simulink model "CMU_BORG_AplysiaModularNeuromechanics"  (R2024a)
settings: Solver=ode23  StartTime=0.0  StopTime=tend  FixedStep=0.001  MaxStep=0.1  RelTol=0.00001  AbsTol=0.0001
values from neighbouring files (symbols this model uses):
  B20_0 = 0    [ParameterRecalculation.m]    (also in ReferenceGeometry_and_Initialization.m)
  B31B32_0 = 0    [GetSteadyState.m]    (also in ParameterRecalculation.m = 1; ReferenceGeometry_and_Initialization.m = 1; VaryingSeaweedStrength.m = 1)
  B38_0 = 0    [ParameterRecalculation.m]    (also in ReferenceGeometry_and_Initialization.m)
  B40B30_0 = 0    [ParameterRecalculation.m]    (also in ReferenceGeometry_and_Initialization.m)
  B40B30_offTime_0 = 0    [ParameterRecalculation.m]    (also in ReferenceGeometry_and_Initialization.m)
  B43B45_0 = 0    [ParameterRecalculation.m]    (also in ReferenceGeometry_and_Initialization.m)
  B4B5_0 = 0    [ParameterRecalculation.m]    (also in ReferenceGeometry_and_Initialization.m)
  B64_0 = 1    [GetSteadyState.m]    (also in ParameterRecalculation.m = 0; ReferenceGeometry_and_Initialization.m = 0; VaryingSeaweedStrength.m = 0)
  B6B9B3_0 = 1    [GetSteadyState.m]    (also in ParameterRecalculation.m = 0; ReferenceGeometry_and_Initialization.m = 0; VaryingSeaweedStrength.m = 0)
  B7_0 = 0    [ParameterRecalculation.m]    (also in ReferenceGeometry_and_Initialization.m)
  B8_0 = 0    [ParameterRecalculation.m]    (also in ReferenceGeometry_and_Initialization.m)
  C1_0 = 0    [ParameterRecalculation.m]    (also in ReferenceGeometry_and_Initialization.m)
  C2_0 = 0    [ParameterRecalculation.m]    (also in ReferenceGeometry_and_Initialization.m)
  C6_0 = 0    [ParameterRecalculation.m]    (also in ReferenceGeometry_and_Initialization.m)
  C_theta = C_xg/(2*pi)    [ParameterRecalculation.m]    (also in ReferenceGeometry_and_Initialization.m = 0.000813600069086)
  C_xd = C_xg    [ParameterRecalculation.m]    (also in ReferenceGeometry_and_Initialization.m = 0.005112)
  C_xg = (1/inv_C(kk))*time_scaler*force_scaler    [DampingParameterConvergence.m]    (also in ReferenceGeometry_and_Initialization.m = 0.005112)
  C_xv = C_xd    [ParameterRecalculation.m]    (also in ReferenceGeometry_and_Initialization.m = 0.005112)
  C_yg = C_xg    [ParameterRecalculation.m]    (also in ReferenceGeometry_and_Initialization.m = 0.005112)
  CBI2_0 = 0    [ParameterRecalculation.m]    (also in ReferenceGeometry_and_Initialization.m)
  CBI3_0 = 0    [GetSteadyState.m]    (also in ParameterRecalculation.m = 1; ReferenceGeometry_and_Initialization.m = 1; VaryingSeaweedStrength.m = 1)
  CBI3_refractory_0 = 0    [ParameterRecalculation.m]    (also in ReferenceGeometry_and_Initialization.m)
  CBI3_stimOFF_0 = 0    [ParameterRecalculation.m]    (also in ReferenceGeometry_and_Initialization.m)
  CBI3_stimON_0 = 0    [ParameterRecalculation.m]    (also in ReferenceGeometry_and_Initialization.m)
  CBI4_0 = 0    [ParameterRecalculation.m]    (also in ReferenceGeometry_and_Initialization.m)
  E1_params = [AE10,TE10,tau_E1,L0_E1,Lmax_E1]    [ParameterRecalculation.m]    (also in ReferenceGeometry_and_Initialization.m)
  E2_params = [AE20,TE20,tau_E2,L0_E2,Lmax_E2]    [ParameterRecalculation.m]    (also in ReferenceGeometry_and_Initialization.m)
  E6_params = [AE60,TE60,tau_E6,L0_E6,Lmax_E6]    [ParameterRecalculation.m]    (also in ReferenceGeometry_and_Initialization.m)
  FE1_max = force_scaler*0.2    [ParameterRecalculation.m]    (also in ReferenceGeometry_and_Initialization.m = 0.048)
  FE2_max = FE1_max    [ParameterRecalculation.m]    (also in ReferenceGeometry_and_Initialization.m = 0.048)
  FE6_max = FE1_max    [ParameterRecalculation.m]    (also in ReferenceGeometry_and_Initialization.m = 0.048)
  FHinge_max = force_scaler*0.292    [ParameterRecalculation.m]    (also in ReferenceGeometry_and_Initialization.m = 0.07008)
  FI1d_max = force_scaler*3.2    [ParameterRecalculation.m]    (also in ReferenceGeometry_and_Initialization.m = 0.768)
  FI1v_max = FI1d_max    [ParameterRecalculation.m]    (also in ReferenceGeometry_and_Initialization.m = 0.768)
  FI2_max = force_scaler*1    [ParameterRecalculation.m]    (also in ReferenceGeometry_and_Initialization.m = 0.24)
  FI3_ant_max = force_scaler*0.1    [ParameterRecalculation.m]    (also in ReferenceGeometry_and_Initialization.m = 0.024)
  FI3_max = force_scaler*3    [ParameterRecalculation.m]    (also in ReferenceGeometry_and_Initialization.m = 0.72)
  FI4_max = force_scaler*0.9    [ParameterRecalculation.m]    (also in ReferenceGeometry_and_Initialization.m = 0.216)
  fixation_type = 0    [GetSteadyState.m]    (also in ModelController.m; VaryingSeaweedStrength.m)
  grasperR = 1    [ReferenceGeometry_and_Initialization.m]
  H_lumen = mean([L_jaw,L_LG]) / R_ref    [ReferenceGeometry_and_Initialization.m]
  Hinge_params = [A_hinge0,T_hinge0,tau_hinge,L0_hinge,Lmax_hinge]    [ParameterRecalculation.m]    (also in ReferenceGeometry_and_Initialization.m)
  I1d_params = [AI1d0,TI1d0,tau_I1d,L0_I1d,Lmax_I1d]    [ParameterRecalculation.m]    (also in ReferenceGeometry_and_Initialization.m)
  I1v_params = [AI1v0,TI1v0,tau_I1v,L0_I1v,Lmax_I1v]    [ParameterRecalculation.m]    (also in ReferenceGeometry_and_Initialization.m)
  I2_params = [AI20,TI20,tau_I2_ingestive,tau_I2_egestive,L0_I2,Lmax_I2]    [ParameterRecalculation.m]    (also in ReferenceGeometry_and_Initialization.m)
  I3_params = [AI30,TI30,tau_I3]    [ParameterRecalculation.m]    (also in ReferenceGeometry_and_Initialization.m)
  I3ant_params = [AI3_ant0,TI3_ant0,tau_I3ant]    [ParameterRecalculation.m]    (also in ReferenceGeometry_and_Initialization.m)
  I4_params = [AI40,TI40,tau_I4]    [ParameterRecalculation.m]    (also in ReferenceGeometry_and_Initialization.m)
  K_const = force_scaler*0.5    [ParameterRecalculation.m]    (also in ReferenceGeometry_and_Initialization.m = 0.12)
  K_Eso = force_scaler*0.01    [ParameterRecalculation.m]    (also in ReferenceGeometry_and_Initialization.m = 0.0024)
  K_H = force_scaler*2    [ParameterRecalculation.m]    (also in ReferenceGeometry_and_Initialization.m = 0.48)
  L0_eso = abs(xd0)    [ReferenceGeometry_and_Initialization.m]
  L0_H = 0    [ReferenceGeometry_and_Initialization.m]
  L0_I1d = L1d0    [ParameterRecalculation.m]    (also in ReferenceGeometry_and_Initialization.m)
  L0_I1v = L1v0    [ParameterRecalculation.m]    (also in ReferenceGeometry_and_Initialization.m)
  L_head = 0.82*tracing_scale_factor    [ReferenceGeometry_and_Initialization.m]
  MCC_0 = 1    [DampingParameterConvergence.m]    (also in ModelController.m; ParameterRecalculation.m = 0; ReferenceGeometry_and_Initialization.m = 0)
  params = param_vec    [ParameterRecalculation.m]    (also in ReferenceGeometry_and_Initialization.m)
  seaweed_strength = 1e6    (= 1000000)    [ModelController.m]    (also in VaryingSeaweedStrength.m = seaweed_strength_vec(ind))
  sens_chemical_lips = 0    [GetSteadyState.m]    (also in ModelController.m = 1; VaryingSeaweedStrength.m = 1)
  sens_mechanical_grasper = 1    [GetSteadyState.m]    (also in ModelController.m = 0; VaryingSeaweedStrength.m)
  sens_mechanical_lips = 1    [GetSteadyState.m]    (also in ModelController.m; VaryingSeaweedStrength.m)
  t_switch_chem_lips = 1e6    (= 1000000)    [GetSteadyState.m]    (also in ModelController.m = 54; VaryingSeaweedStrength.m)
  t_switch_fixation = 1e6    (= 1000000)    [GetSteadyState.m]    (also in ModelController.m = 30; VaryingSeaweedStrength.m = 4)
  t_switch_mech_grasp = 1e6    (= 1000000)    [GetSteadyState.m]    (also in ModelController.m = 10; VaryingSeaweedStrength.m)
  t_switch_mech_lips = 1e6    (= 1000000)    [GetSteadyState.m]    (also in ModelController.m; VaryingSeaweedStrength.m)
  theta_fg = buccal_mass_data(7)    [PlotModel.m]    (also in ReferenceGeometry_and_Initialization.m = -(head_outline{4,"Angle"} - head_outline{3,"Angle"})*(pi/180)
  theta_g0 = (180-(head_outline{3,"Angle"} + rot_global +5))*(pi/180)    [ReferenceGeometry_and_Initialization.m]
  theta_H = buccal_mass_data(6)    [PlotModel.m]    (also in ReferenceGeometry_and_Initialization.m = pi + theta_H_tilde - theta_g0)
  time_scaler = 1    [DampingParameterConvergence.m]    (also in ReferenceGeometry_and_Initialization.m = 1.065)
  ukg = 0.95*usg    (= 0.95)    [ParameterRecalculation.m]    (also in ReferenceGeometry_and_Initialization.m)
  ukh = 0.75*ush    (= 0.75)    [ParameterRecalculation.m]    (also in ReferenceGeometry_and_Initialization.m)
  usg = 1    [ParameterRecalculation.m]    (also in ReferenceGeometry_and_Initialization.m)
  ush = 1    [ParameterRecalculation.m]    (also in ReferenceGeometry_and_Initialization.m)
  xd0 = L_head - L1d0    [ReferenceGeometry_and_Initialization.m]
  xg0 = L_head + L_CG * cosd(a_CG) + 0.3    [ReferenceGeometry_and_Initialization.m]
  xh0 = 0    [ReferenceGeometry_and_Initialization.m]
  xv0 = L_head - L1v0    [ReferenceGeometry_and_Initialization.m]
  yg0 = L_CG * sind(a_CG) + 0.4    [ReferenceGeometry_and_Initialization.m]
(part 3 of 4)

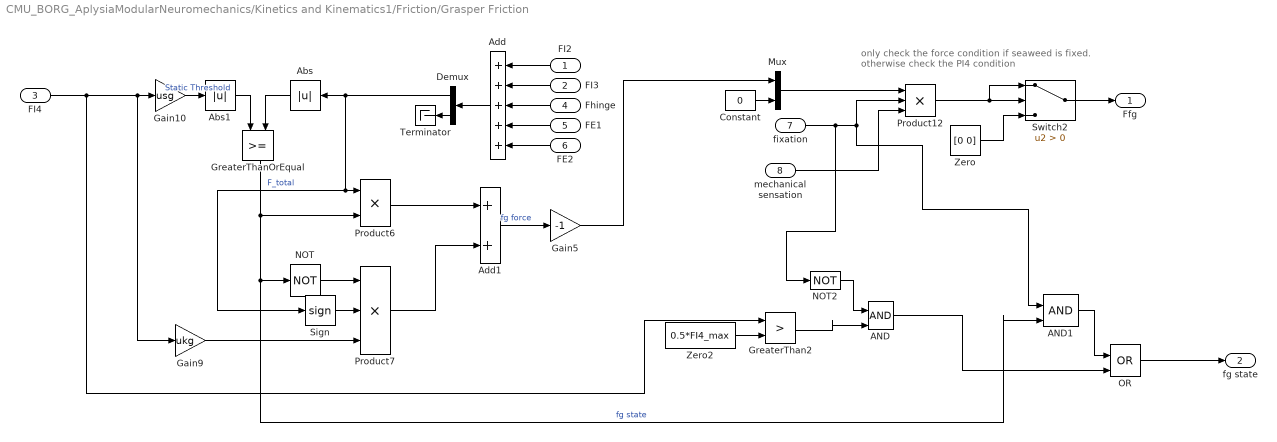
== system CMU_BORG_AplysiaModularNeuromechanics/Kinetics and Kinematics1/Friction/Grasper Friction ==
  note: only check the force condition if seaweed is fixed.
      | otherwise check the PI4 condition
  FI2 : Inport
  FI3 : Inport  Port=2
  FI4 : Inport  Port=3
  Fhinge : Inport  Port=4
  FE1 : Inport  Port=5
  FE2 : Inport  Port=6
  fixation : Inport  Port=7
  mechanical sensation : Inport  Port=8
  AND : Logic  IconShape=distinctive  AllPortsSameDT=off  OutDataTypeStr=boolean
  AND1 : Logic  IconShape=distinctive  AllPortsSameDT=off  OutDataTypeStr=boolean
  Abs : Abs  ZeroCross=off  SaturateOnIntegerOverflow=off
  Abs1 : Abs  ZeroCross=off  SaturateOnIntegerOverflow=off
  Add : Sum  Inputs=+++++
  Add1 : Sum
  Constant : Constant  Value=0
  Demux : Demux  Outputs=2
  Gain10 : Gain  Gain=usg
  Gain5 : Gain  Gain=-1
  Gain9 : Gain  Gain=ukg
  GreaterThan2 : RelationalOperator  Operator=>  OutDataTypeStr=boolean  RndMeth=Simplest  InputSameDT=off
  GreaterThanOrEqual : RelationalOperator  OutDataTypeStr=boolean  ZeroCross=off  RndMeth=Simplest  InputSameDT=off
  Mux : Mux  Inputs=2
  NOT : Logic  Operator=NOT  IconShape=distinctive  AllPortsSameDT=off  OutDataTypeStr=boolean
  NOT2 : Logic  Operator=NOT  IconShape=distinctive  AllPortsSameDT=off  OutDataTypeStr=boolean
  OR : Logic  Operator=OR  IconShape=distinctive  AllPortsSameDT=off  OutDataTypeStr=boolean
  Product12 : Product  Inputs=3
  Product6 : Product
  Product7 : Product  Inputs=3
  Sign : Signum  ZeroCross=off
  Switch2 : Switch  Criteria=u2 > Threshold  SaturateOnIntegerOverflow=off  InputSameDT=off
  Terminator : Terminator
  Zero : Constant  Value=[0 0]  OutDataTypeStr=Inherit: Inherit via back propagation
  Zero2 : Constant  Value=0.5*FI4_max  OutDataTypeStr=Inherit: Inherit via back propagation
  Ffg : Outport
  fg state : Outport  Port=2
  wires:
  Product6/1 -> Add1/1
  Abs1/1 -> GreaterThanOrEqual/1
  NOT/1 -> Product7/1
  Gain9/1 -> Product7/3
  Product7/1 -> Add1/2
  Sign/1 -> Product7/2
  Add1/1 -> Gain5/1  "fg force"
  Abs/1 -> GreaterThanOrEqual/2
  FI4/1 -> GreaterThan2/1, Gain10/1, Gain9/1
  GreaterThanOrEqual/1 -> AND1/2, NOT/1, Product6/2  "fg state"
  Gain10/1 -> Abs1/1  "Static Threshold"
  FI2/1 -> Add/1
  FE2/1 -> Add/5
  FE1/1 -> Add/4
  Fhinge/1 -> Add/3
  FI3/1 -> Add/2
  Add/1 -> Demux/1
  Demux/1 -> Sign/1, Product6/1, Abs/1  "F_total"
  Demux/2 -> Terminator/1
  Constant/1 -> Mux/2
  mechanical sensation/1 -> Product12/3
  fixation/1 -> NOT2/1, AND1/1, Product12/2
  Mux/1 -> Product12/1
  Product12/1 -> Switch2/2, Switch2/1
  Zero/1 -> Switch2/3
  Switch2/1 -> Ffg/1
  Gain5/1 -> Mux/1
  OR/1 -> fg state/1
  AND/1 -> OR/2
  Zero2/1 -> GreaterThan2/2
  AND1/1 -> OR/1
  GreaterThan2/1 -> AND/2
  NOT2/1 -> AND/1

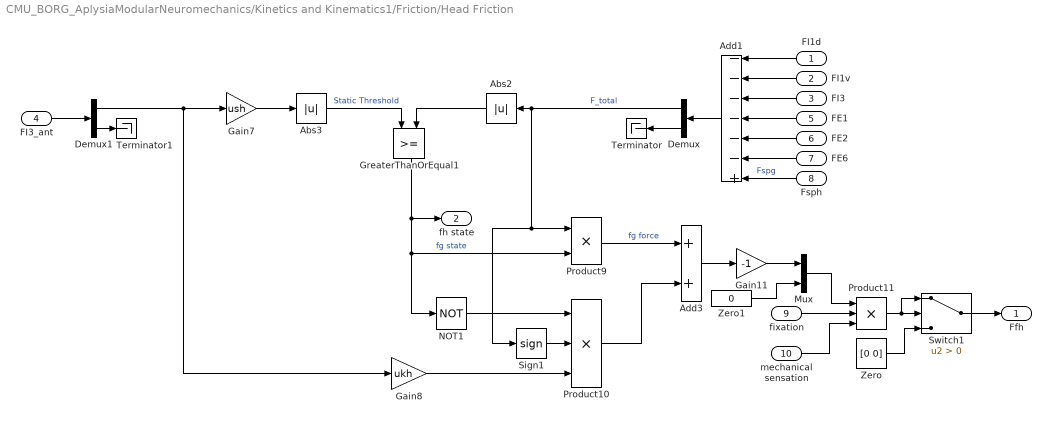
== system CMU_BORG_AplysiaModularNeuromechanics/Kinetics and Kinematics1/Friction/Head Friction ==
  FI1d : Inport
  FI1v : Inport  Port=2
  FI3 : Inport  Port=3
  FI3_ant : Inport  Port=4
  FE1 : Inport  Port=5
  FE2 : Inport  Port=6
  FE6 : Inport  Port=7
  Fsph : Inport  Port=8
  fixation : Inport  Port=9
  mechanical sensation : Inport  Port=10
  Abs2 : Abs  ZeroCross=off  SaturateOnIntegerOverflow=off
  Abs3 : Abs  ZeroCross=off  SaturateOnIntegerOverflow=off
  Add1 : Sum  Inputs=------+
  Add3 : Sum
  Demux : Demux  Outputs=2
  Demux1 : Demux  Outputs=2
  Gain11 : Gain  Gain=-1
  Gain7 : Gain  Gain=ush
  Gain8 : Gain  Gain=ukh
  GreaterThanOrEqual1 : RelationalOperator  OutDataTypeStr=boolean  ZeroCross=off  RndMeth=Simplest  InputSameDT=off
  Mux : Mux  Inputs=2
  NOT1 : Logic  Operator=NOT  IconShape=distinctive  AllPortsSameDT=off  OutDataTypeStr=boolean
  Product10 : Product  Inputs=3
  Product11 : Product  Inputs=3
  Product9 : Product
  Sign1 : Signum  ZeroCross=off
  Switch1 : Switch  Criteria=u2 > Threshold  SaturateOnIntegerOverflow=off  InputSameDT=off
  Terminator : Terminator
  Terminator1 : Terminator
  Zero : Constant  Value=[0 0]  OutDataTypeStr=Inherit: Inherit via back propagation
  Zero1 : Constant  Value=0  OutDataTypeStr=Inherit: Inherit via back propagation
  Ffh : Outport
  fh state : Outport  Port=2
  wires:
  Add3/1 -> Gain11/1
  Gain8/1 -> Product10/3
  Product10/1 -> Add3/2
  Gain7/1 -> Abs3/1
  NOT1/1 -> Product10/1
  Sign1/1 -> Product10/2
  Abs2/1 -> GreaterThanOrEqual1/2
  FI1d/1 -> Add1/1
  FI1v/1 -> Add1/2
  FI3/1 -> Add1/3
  FE1/1 -> Add1/4
  FE2/1 -> Add1/5
  FE6/1 -> Add1/6
  Fsph/1 -> Add1/7  "Fspg"
  Add1/1 -> Demux/1
  Demux/2 -> Terminator/1
  fixation/1 -> Product11/2
  mechanical sensation/1 -> Product11/3
  Product11/1 -> Switch1/2, Switch1/1
  Zero/1 -> Switch1/3
  Product9/1 -> Add3/1  "fg force"
  Abs3/1 -> GreaterThanOrEqual1/1  "Static Threshold"
  GreaterThanOrEqual1/1 -> NOT1/1, Product9/2, fh state/1  "fg state"
  Demux/1 -> Sign1/1, Product9/1, Abs2/1  "F_total"
  Demux1/1 -> Gain8/1, Gain7/1
  FI3_ant/1 -> Demux1/1
  Demux1/2 -> Terminator1/1
  Gain11/1 -> Mux/1
  Mux/1 -> Product11/1
  Zero1/1 -> Mux/2
  Switch1/1 -> Ffh/1

== system CMU_BORG_AplysiaModularNeuromechanics/Kinetics and Kinematics1/Kinematics (Circular Odontophore)/E1 Length//Angle ==
  Anchor : Inport
  Attachment : Inport  Port=2
  Add : Sum
  Atan : Trigonometry  Operator=atan
  Demux1 : Demux  Outputs=2
  Demux3 : Demux  Outputs=2
  Divide : Product  Inputs=/*
  Sqrt : Sqrt
  Square : Math  Operator=square
  Sum3 : Sum  Inputs=+-|
  L : Outport
  phi : Outport  Port=2
  wires:
  Add/1 -> Sqrt/1
  Square/1 -> Demux3/1
  Demux3/2 -> Add/2
  Demux3/1 -> Add/1
  Sum3/1 -> Demux1/1, Square/1
  Anchor/1 -> Sum3/1
  Attachment/1 -> Sum3/2
  Sqrt/1 -> L/1
  Demux1/1 -> Divide/1
  Demux1/2 -> Divide/2
  Divide/1 -> Atan/1
  Atan/1 -> phi/1

== system CMU_BORG_AplysiaModularNeuromechanics/Kinetics and Kinematics1/Kinematics (Circular Odontophore)/E2 Length//Angle ==
  Anchor : Inport
  Attachment : Inport  Port=2
  Add : Sum
  Atan : Trigonometry  Operator=atan
  Demux1 : Demux  Outputs=2
  Demux3 : Demux  Outputs=2
  Divide : Product  Inputs=/*
  Sqrt : Sqrt
  Square : Math  Operator=square
  Sum3 : Sum  Inputs=+-|
  L : Outport
  phi : Outport  Port=2
  wires:
  Atan/1 -> phi/1
  Divide/1 -> Atan/1
  Demux1/2 -> Divide/2
  Demux1/1 -> Divide/1
  Sqrt/1 -> L/1
  Attachment/1 -> Sum3/2
  Anchor/1 -> Sum3/1
  Sum3/1 -> Square/1, Demux1/1
  Demux3/1 -> Add/1
  Demux3/2 -> Add/2
  Square/1 -> Demux3/1
  Add/1 -> Sqrt/1

== system CMU_BORG_AplysiaModularNeuromechanics/Kinetics and Kinematics1/Kinematics (Circular Odontophore)/E6 Length//Angle ==
  Anchor : Inport  PortDimensions=2
  Attachment : Inport  Port=2
  Add : Sum
  Atan : Trigonometry  Operator=atan
  Demux1 : Demux  Outputs=2
  Demux3 : Demux  Outputs=2
  Divide : Product  Inputs=/*
  Sqrt : Sqrt
  Square : Math  Operator=square
  Sum3 : Sum  Inputs=+-|
  L : Outport
  phi : Outport  Port=2
  wires:
  Atan/1 -> phi/1
  Divide/1 -> Atan/1
  Demux1/2 -> Divide/2
  Demux1/1 -> Divide/1
  Sqrt/1 -> L/1
  Attachment/1 -> Sum3/2
  Anchor/1 -> Sum3/1
  Sum3/1 -> Square/1, Demux1/1
  Demux3/1 -> Add/1
  Demux3/2 -> Add/2
  Square/1 -> Demux3/1
  Add/1 -> Sqrt/1

== system CMU_BORG_AplysiaModularNeuromechanics/Kinetics and Kinematics1/Kinematics (Circular Odontophore)/Hinge Length//Angle ==
  Attachment : Inport
  Anchor : Inport  Port=2
  Add : Sum
  Atan : Trigonometry  Operator=atan
  Constant : Constant  Value=0
  Demux1 : Demux  Outputs=2
  Demux3 : Demux  Outputs=2
  Divide : Product  Inputs=/*
  Sqrt : Sqrt
  Square : Math  Operator=square
  Sum3 : Sum  Inputs=+-|
  L : Outport
  phi : Outport  Port=2
  wires:
  Divide/1 -> Atan/1
  Demux1/2 -> Divide/2
  Demux1/1 -> Divide/1
  Attachment/1 -> Sum3/2
  Anchor/1 -> Sum3/1
  Sum3/1 -> Square/1, Demux1/1
  Demux3/1 -> Add/1
  Square/1 -> Demux3/1
  Add/1 -> Sqrt/1
  Sqrt/1 -> L/1
  Atan/1 -> phi/1
  Constant/1 -> Add/2

== system CMU_BORG_AplysiaModularNeuromechanics/Kinetics and Kinematics1/Kinematics (Circular Odontophore)/I1d Length//Angle ==
  Anchor : Inport
  Attachment : Inport  Port=2
  Add : Sum
  Atan : Trigonometry  Operator=atan
  Demux1 : Demux  Outputs=2
  Demux3 : Demux  Outputs=2
  Divide : Product  Inputs=/*
  Sqrt : Sqrt
  Square : Math  Operator=square
  Sum3 : Sum  Inputs=+-|
  L : Outport
  phi : Outport  Port=2
  wires:
  Atan/1 -> phi/1
  Divide/1 -> Atan/1
  Demux1/2 -> Divide/2
  Demux1/1 -> Divide/1
  Sqrt/1 -> L/1
  Attachment/1 -> Sum3/2
  Anchor/1 -> Sum3/1
  Sum3/1 -> Square/1, Demux1/1
  Demux3/1 -> Add/1
  Demux3/2 -> Add/2
  Square/1 -> Demux3/1
  Add/1 -> Sqrt/1

== system CMU_BORG_AplysiaModularNeuromechanics/Kinetics and Kinematics1/Kinematics (Circular Odontophore)/I1v Length//Angle ==
  Anchor : Inport
  Attachment : Inport  Port=2
  Add : Sum
  Atan : Trigonometry  Operator=atan
  Demux1 : Demux  Outputs=2
  Demux3 : Demux  Outputs=2
  Divide : Product  Inputs=/*
  Sqrt : Sqrt
  Square : Math  Operator=square
  Sum3 : Sum  Inputs=+-|
  L : Outport
  phi : Outport  Port=2
  wires:
  Add/1 -> Sqrt/1
  Square/1 -> Demux3/1
  Demux3/2 -> Add/2
  Demux3/1 -> Add/1
  Sum3/1 -> Demux1/1, Square/1
  Anchor/1 -> Sum3/1
  Attachment/1 -> Sum3/2
  Sqrt/1 -> L/1
  Demux1/1 -> Divide/1
  Demux1/2 -> Divide/2
  Divide/1 -> Atan/1
  Atan/1 -> phi/1

== system CMU_BORG_AplysiaModularNeuromechanics/Kinetics and Kinematics1/Kinematics (Circular Odontophore)/I2d Length//Angle ==
  Anchor : Inport
  Attachment : Inport  Port=2
  Add : Sum
  Atan : Trigonometry  Operator=atan
  Demux1 : Demux  Outputs=2
  Demux3 : Demux  Outputs=2
  Divide : Product  Inputs=/*
  Sqrt : Sqrt
  Square : Math  Operator=square
  Sum3 : Sum  Inputs=+-|
  L : Outport
  phi : Outport  Port=2
  wires:
  Atan/1 -> phi/1
  Divide/1 -> Atan/1
  Demux1/2 -> Divide/2
  Demux1/1 -> Divide/1
  Sqrt/1 -> L/1
  Attachment/1 -> Sum3/2
  Anchor/1 -> Sum3/1
  Sum3/1 -> Square/1, Demux1/1
  Demux3/1 -> Add/1
  Demux3/2 -> Add/2
  Square/1 -> Demux3/1
  Add/1 -> Sqrt/1

== system CMU_BORG_AplysiaModularNeuromechanics/Kinetics and Kinematics1/Kinematics (Circular Odontophore)/I2v Length//Angle1 ==
  note: Switch accounts for when hinge is inside odontophore. If inside,
      | state that the I2 angle is 0 relative to the horizontal.
  Attachment : Inport
  Anchor : Inport  Port=2
  Add : Sum
  Atan : Trigonometry  Operator=atan
  Constant : Constant  Value=0
  Demux1 : Demux  Outputs=2
  Demux3 : Demux  Outputs=2
  Divide : Product  Inputs=/*
  Sqrt : Sqrt
  Square : Math  Operator=square
  Sum3 : Sum  Inputs=+-|
  Switch : Switch  Criteria=u2 > Threshold  SaturateOnIntegerOverflow=off  InputSameDT=off
  phi : Outport
  L : Outport  Port=2
  wires:
  Add/1 -> Sqrt/1
  Square/1 -> Demux3/1
  Demux3/2 -> Add/2
  Demux3/1 -> Add/1
  Sum3/1 -> Demux1/1, Square/1
  Anchor/1 -> Sum3/1
  Attachment/1 -> Sum3/2
  Sqrt/1 -> L/1
  Divide/1 -> Atan/1
  Demux1/2 -> Divide/2
  Demux1/1 -> Divide/1, Switch/2
  Constant/1 -> Switch/3
  Switch/1 -> phi/1
  Atan/1 -> Switch/1

== system CMU_BORG_AplysiaModularNeuromechanics/Kinetics and Kinematics1/Kinematics (Circular Odontophore)/Length//Angle Template ==
  Anchor : Inport
  Attachment : Inport  Port=2
  Add : Sum
  Atan : Trigonometry  Operator=atan
  Demux1 : Demux  Outputs=2
  Demux3 : Demux  Outputs=2
  Divide : Product  Inputs=/*
  Sqrt : Sqrt
  Square : Math  Operator=square
  Sum3 : Sum  Inputs=+-|
  L : Outport
  phi : Outport  Port=2
  wires:
  Add/1 -> Sqrt/1
  Square/1 -> Demux3/1
  Demux3/2 -> Add/2
  Demux3/1 -> Add/1
  Sum3/1 -> Demux1/1, Square/1
  Anchor/1 -> Sum3/1
  Attachment/1 -> Sum3/2
  Sqrt/1 -> L/1
  Demux1/1 -> Divide/1
  Demux1/2 -> Divide/2
  Divide/1 -> Atan/1
  Atan/1 -> phi/1

== system CMU_BORG_AplysiaModularNeuromechanics/Kinetics and Kinematics1/Muscles Mechanical Advantage Module/E1 Force Deccomposition ==
  T : Inport
  phi : Inport  Port=2
  Cos : Trigonometry  Operator=cos
  Cos1 : Trigonometry
  Mux : Mux  Inputs=2
  Product : Product
  F : Outport
  wires:
  phi/1 -> Cos/1, Cos1/1
  Cos/1 -> Mux/1
  Cos1/1 -> Mux/2
  Product/1 -> F/1
  T/1 -> Product/2
  Mux/1 -> Product/1

== system CMU_BORG_AplysiaModularNeuromechanics/Kinetics and Kinematics1/Muscles Mechanical Advantage Module/E2 Force Decomposition ==
  T : Inport
  phi : Inport  Port=2
  Cos : Trigonometry  Operator=cos
  Cos1 : Trigonometry
  Mux : Mux  Inputs=2
  Product : Product
  F : Outport
  wires:
  Mux/1 -> Product/1
  T/1 -> Product/2
  Product/1 -> F/1
  Cos1/1 -> Mux/2
  Cos/1 -> Mux/1
  phi/1 -> Cos1/1, Cos/1

== system CMU_BORG_AplysiaModularNeuromechanics/Kinetics and Kinematics1/Muscles Mechanical Advantage Module/E6 ForceDecomposition ==
  T : Inport
  phi : Inport  Port=2
  Cos : Trigonometry  Operator=cos
  Cos1 : Trigonometry
  Mux : Mux  Inputs=2
  Product : Product
  F : Outport
  wires:
  phi/1 -> Cos/1, Cos1/1
  Cos/1 -> Mux/1
  Cos1/1 -> Mux/2
  Product/1 -> F/1
  T/1 -> Product/2
  Mux/1 -> Product/1

== system CMU_BORG_AplysiaModularNeuromechanics/Kinetics and Kinematics1/Muscles Mechanical Advantage Module/Force Vector Decomposition Template ==
  T : Inport
  phi : Inport  Port=2
  Cos : Trigonometry  Operator=cos
  Cos1 : Trigonometry
  Mux : Mux  Inputs=2
  Product : Product
  F : Outport
  wires:
  phi/1 -> Cos/1, Cos1/1
  Cos/1 -> Mux/1
  Cos1/1 -> Mux/2
  Product/1 -> F/1
  T/1 -> Product/2
  Mux/1 -> Product/1

== system CMU_BORG_AplysiaModularNeuromechanics/Kinetics and Kinematics1/Muscles Mechanical Advantage Module/Hinge Force Decomposition ==
  T : Inport
  phi : Inport  Port=2
  Constant : Constant
  Cos : Trigonometry  Operator=cos
  Cos1 : Trigonometry
  Mux : Mux  Inputs=2
  Product : Product
  Terminator : Terminator
  F : Outport
  wires:
  phi/1 -> Cos/1, Cos1/1
  Cos/1 -> Mux/1
  Cos1/1 -> Mux/2
  Product/1 -> F/1
  T/1 -> Product/2
  Constant/1 -> Product/1
  Mux/1 -> Terminator/1

== system CMU_BORG_AplysiaModularNeuromechanics/Kinetics and Kinematics1/Muscles Mechanical Advantage Module/I1d Force Decomposition ==
  T : Inport
  phi : Inport  Port=2
  Cos : Trigonometry  Operator=cos
  Cos1 : Trigonometry
  Mux : Mux  Inputs=2
  Product : Product
  F : Outport
  wires:
  Mux/1 -> Product/1
  T/1 -> Product/2
  Product/1 -> F/1
  Cos1/1 -> Mux/2
  Cos/1 -> Mux/1
  phi/1 -> Cos1/1, Cos/1

== system CMU_BORG_AplysiaModularNeuromechanics/Kinetics and Kinematics1/Muscles Mechanical Advantage Module/I1v Force Decomposition ==
  T : Inport
  phi : Inport  Port=2
  Cos : Trigonometry  Operator=cos
  Cos1 : Trigonometry
  Mux : Mux  Inputs=2
  Product : Product
  F : Outport
  wires:
  phi/1 -> Cos/1, Cos1/1
  Cos/1 -> Mux/1
  Cos1/1 -> Mux/2
  Product/1 -> F/1
  T/1 -> Product/2
  Mux/1 -> Product/1

== system CMU_BORG_AplysiaModularNeuromechanics/Kinetics and Kinematics1/Muscles Mechanical Advantage Module/I3 ==
  TI3 : Inport
  xg : Inport  Port=2
  xv : Inport  Port=3
  xd : Inport  Port=4
  xh : Inport  Port=5
  Constant : Constant  Value=0
  Constant2 : Constant  Value=grasperR
  Constant3 : Constant  Value=L_head
  Gain : Gain  Gain=-1
  MATLAB Function : MATLAB Function  TreatAsAtomicUnit=on
  Mux : Mux  Inputs=2
  Product4 : Product
  FI3 : Outport
  wires:
  Product4/1 -> Mux/1  "FI3"
  Mux/1 -> Gain/1
  Constant/1 -> Mux/2
  Gain/1 -> FI3/1
  xg/1 -> MATLAB Function/2(xg)
  xv/1 -> MATLAB Function/3(xv)
  xd/1 -> MATLAB Function/4(xd)
  Constant2/1 -> MATLAB Function/5(R)
  xh/1 -> MATLAB Function/1(xh)
  Constant3/1 -> MATLAB Function/6(L_head)
  TI3/1 -> Product4/2
  MATLAB Function/1(MA) -> Product4/1

== system CMU_BORG_AplysiaModularNeuromechanics/Kinetics and Kinematics1/Muscles Mechanical Advantage Module/I3_ant ==
  TI3 : Inport
  Constant : Constant  Value=0
  Gain : Gain
  Mux : Mux  Inputs=2
  One : Constant  OutDataTypeStr=Inherit: Inherit via back propagation
  Product4 : Product
  FI3 : Outport
  wires:
  Gain/1 -> FI3/1
  Constant/1 -> Mux/2
  Mux/1 -> Gain/1
  TI3/1 -> Product4/2
  One/1 -> Product4/1
  Product4/1 -> Mux/1  "FI3"

== system CMU_BORG_AplysiaModularNeuromechanics/Kinetics and Kinematics1/Muscles Mechanical Advantage Module/Subsystem ==
  TI2 : Inport
  phi_I2d : Inport  Port=2
  phi_I2v : Inport  Port=3
  Gain : Gain  Gain=-1
  Gain1 : Gain  Gain=-1
  Mux : Mux  Inputs=2
  Mux1 : Mux  Inputs=2
  Product : Product
  Product1 : Product
  Sin : Trigonometry
  Sin1 : Trigonometry  Operator=cos
  Sin2 : Trigonometry
  Sin3 : Trigonometry  Operator=cos
  FI2_d : Outport
  FI2_v : Outport  Port=2
  wires:
  phi_I2v/1 -> Sin3/1, Sin2/1
  phi_I2d/1 -> Sin1/1, Sin/1
  Mux/1 -> Product/1
  Product/1 -> FI2_d/1
  Mux1/1 -> Product1/2
  Product1/1 -> FI2_v/1
  TI2/1 -> Product1/1, Product/2
  Sin/1 -> Mux/1
  Gain/1 -> Mux/2
  Sin1/1 -> Gain/1
  Sin2/1 -> Gain1/1
  Sin3/1 -> Mux1/2
  Gain1/1 -> Mux1/1

== system CMU_BORG_AplysiaModularNeuromechanics/Kinetics and Kinematics1/Springs/Esophagus Spring ==
  xd : Inport
  Constant4 : Constant  Value=L0_eso
  Gain : Gain  Gain=-1
  Kg : Gain  Gain=K_Eso
  Mux : Mux  Inputs=2
  Sum5 : Sum  Inputs=+-|
  Switch : Switch  Criteria=u2 > Threshold  SaturateOnIntegerOverflow=off  InputSameDT=off
  Zero : Constant  Value=0  OutDataTypeStr=Inherit: Inherit via back propagation
  F_eso : Outport
  wires:
  xd/1 -> Sum5/1
  Kg/1 -> Switch/1  "Fspg_z"
  Sum5/1 -> Kg/1, Switch/2
  Constant4/1 -> Sum5/2
  Switch/1 -> Gain/1
  Zero/1 -> Mux/2, Switch/3
  Mux/1 -> F_eso/1
  Gain/1 -> Mux/1

== system CMU_BORG_AplysiaModularNeuromechanics/Kinetics and Kinematics1/Springs/Grasper-Head Spring1 ==
  xh : Inport
  Constant4 : Constant  Value=L0_H
  Gain : Gain  Gain=-1
  K : Gain  Gain=K_H
  Mux : Mux  Inputs=2
  Sum5 : Sum  Inputs=+-|
  Zero : Constant  Value=0  OutDataTypeStr=Inherit: Inherit via back propagation
  F_sph : Outport
  wires:
  Gain/1 -> Mux/1
  Mux/1 -> F_sph/1
  Zero/1 -> Mux/2
  K/1 -> Gain/1
  Constant4/1 -> Sum5/2
  Sum5/1 -> K/1
  xh/1 -> Sum5/1

== system CMU_BORG_AplysiaModularNeuromechanics/Kinetics and Kinematics1/Equations of Motion/Calculate Sum of Torques/2D Cross Product ==
  a : Inport
  b : Inport  Port=2
  Add : Sum  Inputs=+-
  Demux : Demux  Outputs=2
  Demux1 : Demux  Outputs=2
  Product : Product
  Product1 : Product
  axb : Outport
  wires:
  a/1 -> Demux/1
  b/1 -> Demux1/1
  Demux/1 -> Product/1
  Demux1/2 -> Product/2
  Demux1/1 -> Product1/1
  Demux/2 -> Product1/2
  Add/1 -> axb/1
  Product/1 -> Add/1
  Product1/1 -> Add/2

== system CMU_BORG_AplysiaModularNeuromechanics/Kinetics and Kinematics1/Equations of Motion/Calculate Sum of Torques/2D Cross Product1 ==
  a : Inport
  b : Inport  Port=2
  Add : Sum  Inputs=+-
  Demux : Demux  Outputs=2
  Demux1 : Demux  Outputs=2
  Product : Product
  Product1 : Product
  axb : Outport
  wires:
  Product1/1 -> Add/2
  Product/1 -> Add/1
  Add/1 -> axb/1
  Demux/2 -> Product1/2
  Demux1/1 -> Product1/1
  Demux1/2 -> Product/2
  Demux/1 -> Product/1
  b/1 -> Demux1/1
  a/1 -> Demux/1

== system CMU_BORG_AplysiaModularNeuromechanics/Kinetics and Kinematics1/Equations of Motion/Calculate Sum of Torques/2D Cross Product2 ==
  a : Inport
  b : Inport  Port=2
  Add : Sum  Inputs=+-
  Demux : Demux  Outputs=2
  Demux1 : Demux  Outputs=2
  Product : Product
  Product1 : Product
  axb : Outport
  wires:
  a/1 -> Demux/1
  b/1 -> Demux1/1
  Demux/1 -> Product/1
  Demux1/2 -> Product/2
  Demux1/1 -> Product1/1
  Demux/2 -> Product1/2
  Add/1 -> axb/1
  Product/1 -> Add/1
  Product1/1 -> Add/2

== system CMU_BORG_AplysiaModularNeuromechanics/Kinetics and Kinematics1/Equations of Motion/Calculate Sum of Torques/2D Cross Product3 ==
  a : Inport
  b : Inport  Port=2
  Add : Sum  Inputs=+-
  Demux : Demux  Outputs=2
  Demux1 : Demux  Outputs=2
  Product : Product
  Product1 : Product
  axb : Outport
  wires:
  Product1/1 -> Add/2
  Product/1 -> Add/1
  Add/1 -> axb/1
  Demux/2 -> Product1/2
  Demux1/1 -> Product1/1
  Demux1/2 -> Product/2
  Demux/1 -> Product/1
  b/1 -> Demux1/1
  a/1 -> Demux/1

== system CMU_BORG_AplysiaModularNeuromechanics/Kinetics and Kinematics1/Equations of Motion/Calculate Sum of Torques/2D Cross Product4 ==
  a : Inport
  b : Inport  Port=2
  Add : Sum  Inputs=+-
  Demux : Demux  Outputs=2
  Demux1 : Demux  Outputs=2
  Product : Product
  Product1 : Product
  axb : Outport
  wires:
  a/1 -> Demux/1
  b/1 -> Demux1/1
  Demux/1 -> Product/1
  Demux1/2 -> Product/2
  Demux1/1 -> Product1/1
  Demux/2 -> Product1/2
  Add/1 -> axb/1
  Product/1 -> Add/1
  Product1/1 -> Add/2

== system CMU_BORG_AplysiaModularNeuromechanics/Kinetics and Kinematics1/Equations of Motion/Calculate Sum of Torques/2D Cross Product5 ==
  a : Inport
  b : Inport  Port=2
  Add : Sum  Inputs=+-
  Demux : Demux  Outputs=2
  Demux1 : Demux  Outputs=2
  Product : Product
  Product1 : Product
  axb : Outport
  wires:
  Product1/1 -> Add/2
  Product/1 -> Add/1
  Add/1 -> axb/1
  Demux/2 -> Product1/2
  Demux1/1 -> Product1/1
  Demux1/2 -> Product/2
  Demux/1 -> Product/1
  b/1 -> Demux1/1
  a/1 -> Demux/1

== system CMU_BORG_AplysiaModularNeuromechanics/Kinetics and Kinematics1/Equations of Motion/Calculate Sum of Torques/Constraint Torque ==
  thetag : Inport
  Add : Sum  Inputs=--+
  Constant : Constant  Value=theta_H
  Constant1 : Constant  Value=3*pi/2
  Multiply : Gain  Gain=K_const
  Switch : Switch  Criteria=u2 > Threshold  SaturateOnIntegerOverflow=off  InputSameDT=off
  Zero : Constant  Value=0  OutDataTypeStr=Inherit: Inherit via back propagation
  Constraint Torque : Outport
  wires:
  thetag/1 -> Add/1
  Constant/1 -> Add/2
  Constant1/1 -> Add/3
  Add/1 -> Switch/2, Switch/1
  Zero/1 -> Switch/3
  Switch/1 -> Multiply/1
  Multiply/1 -> Constraint Torque/1

== system CMU_BORG_AplysiaModularNeuromechanics/Kinetics and Kinematics1/Equations of Motion/Calculate Sum of Torques/r_Fg ==
  thetag : Inport
  Constant : Constant  Value=theta_fg
  Cos : Trigonometry  Operator=cos
  Cos1 : Trigonometry
  Gain : Gain  Gain=grasperR
  Mux : Mux  Inputs=2
  Sum : Sum  Inputs=|+-
  r_Fg : Outport
  wires:
  thetag/1 -> Sum/1
  Constant/1 -> Sum/2
  Sum/1 -> Cos/1, Cos1/1
  Cos/1 -> Mux/1
  Mux/1 -> Gain/1
  Gain/1 -> r_Fg/1
  Cos1/1 -> Mux/2

== system CMU_BORG_AplysiaModularNeuromechanics/Kinetics and Kinematics1/Equations of Motion/Calculate Sum of Torques/r_H ==
  thetag : Inport
  Constant : Constant  Value=theta_H
  Cos2 : Trigonometry
  Cos3 : Trigonometry  Operator=cos
  Gain : Gain  Gain=grasperR
  Mux : Mux  Inputs=2
  Sum : Sum  Inputs=|++
  r_H : Outport
  wires:
  Gain/1 -> r_H/1
  Mux/1 -> Gain/1
  Cos3/1 -> Mux/1
  Sum/1 -> Cos2/1, Cos3/1
  Constant/1 -> Sum/2
  thetag/1 -> Sum/1
  Cos2/1 -> Mux/2

== system CMU_BORG_AplysiaModularNeuromechanics/Kinetics and Kinematics1/Equations of Motion/Calculate Sum of Torques/r_I3 ==
  yg : Inport
  Add : Sum  Inputs=+-
  Add2 : Sum  Inputs=+-
  Constant : Constant  Value=H_lumen/2
  Display : Display
  Display1 : Display
  Mux : Mux  Inputs=2
  Sqrt : Sqrt  Operator=signedSqrt
  Square : Math  Operator=square
  grasperR : Constant  Value=grasperR^2
  r_I3 : Outport
  wires:
  Mux/1 -> r_I3/1
  yg/1 -> Add/2
  Constant/1 -> Add/1
  Add/1 -> Display1/1, Mux/2, Square/1
  Sqrt/1 -> Mux/1
  Add2/1 -> Display/1, Sqrt/1
  Square/1 -> Add2/2
  grasperR/1 -> Add2/1

== matlab function CMU_BORG_AplysiaModularNeuromechanics/Muscle Activation and Tension Module/Hinge - First Order + Spring Muscle Model/MATLAB Function ==
  data: L input; T output; L0 input; L_max input; dL output
function [T,dL] = fcn(L,L0,L_max)

%y = 4*( ((L_max/L0) - 1 + (L_max/L0)-1 ) / (L_max - L0) )*( (L0 / L) + (L / L0) - 2 );
T = (L - L0)./(L_max - L0);
dL = L-L0;

== matlab function CMU_BORG_AplysiaModularNeuromechanics/Kinetics and Kinematics1/Equations of Motion/Solving for Lagrange Multiplier/Constraint Derivatives ==
  data: dfdtheta output; yg input; dfdy output; theta_g input; R input; theta_H input
function [dfdtheta,dfdy] = fcn(yg,theta_g,R,theta_H)

% original constraint equation f(y,theta) = y - R sin(theta + theta_H)
dfdy = 1;
dfdtheta = R*cos(theta_g + theta_H);

% quadratic constraint equation f(y,theta) = y^2 - (R cos(theta + % theta_H))^2
%dfdy = 2*yg;
%dfdtheta = -2*(R^2)*cos(theta_g + theta_H)*sin(theta_g+theta_H);

== matlab function CMU_BORG_AplysiaModularNeuromechanics/Neural Model Module Webster-Wood et al. 1/MATLAB Function1 ==
  data: MCC_old input; CBI4_old input; B4B5 input; B82 output; B64_old input; C1 output; C2 output; C6 output; CBI3_old input
function [B82,C1,C2,C6] = AdditionalNeurons(MCC_old,CBI4_old, B4B5, B64_old, CBI3_old)
% Adds additional neurons to innervate the I1, E1, E2, and E6 muscles


% Muscle active during protraction (when B64 is off)

C1 = MCC_old * (~B64_old);
C6 = C1;
B82 = MCC_old * ~((B64_old)); 

% Muscle active during retraction (when B64 is on)

C2 = MCC_old * (B64_old) * (B4B5 < 2);

== matlab function CMU_BORG_AplysiaModularNeuromechanics/Kinetics and Kinematics1/Muscles Mechanical Advantage Module/I3/MATLAB Function ==
  data: xh input; xg input; MA output; xv input; xd input; R input; L_head input; dxp output
function [MA,dxp] = fcn(xh, xg,xv,xd,R, L_head)

dxp = (xg + R) - 0.5*(xd + xv);

if dxp > 2*R
    MA_p = 1;
elseif dxp < 0
    MA_p = 0;
else
    MA_p = dxp / (2*R);
end

MA = MA_p;

== matlab function CMU_BORG_AplysiaModularNeuromechanics/MATLAB Function ==
  data: xg input; xh input; xd input; xv input; R input; L_head input; x_gh output
function x_gh  = fcn(xg,xh,xd,xv,R, L_head)


x_gh = (xg + R) - (L_head + xh); % distance from jaw line

== matlab function CMU_BORG_AplysiaModularNeuromechanics/Kinetics and Kinematics1/I3 Body Wall Contact Force/MATLAB Function ==
  data: xg input; yg input; x_hinge input; xv input; F output; R input
function F  = BodyWallContact(xg, yg, x_hinge, xv, R)

% direction to the center of mass -- for a circle, this is equivalent to
% the force being perpendicular to the edge
r = [xg - xv; yg];
r = r / norm(r);

if(xg > x_hinge)
    % the odontophore is inside the lumen so this doesn't come into play
    F = [0;0];

else
    % odontophore is behind the lumen
    dr = (xg - xv)^2 + yg^2;
    if(dr < R^2)
        % the body wall point is inside the odontophore
        F_mag = 10*sqrt(R^2 - dr); % proportional to the level of interseciton
    else
        F_mag = 0;
    end
    F = F_mag * r;
end

end

== matlab function CMU_BORG_AplysiaModularNeuromechanics/Kinetics and Kinematics1/Seaweed Ingestion Calculations/MATLAB Function ==
  data: dL_ingested output; dxg input; dthetag input; thetag input; dxf output; fg_state input; FI3_ant_norm input; theta_fg input; grasperR input; sense_mechanical_grasper input
function [dL_ingested,dxf] = Length_of_Ingested_Seaweed(dxg,dthetag,thetag,fg_state,FI3_ant_norm,theta_fg,grasperR,sense_mechanical_grasper)

dxf = dxg - grasperR*sin( thetag - theta_fg )*dthetag;

grasper_closed_on_food = fg_state * sense_mechanical_grasper; % is the grasper closed onto food?
pushing_forward = dxf > 0; % is the food moving forward?
jaws_closed = FI3_ant_norm > 0.5; % are the jaws closed to prevent egestion?

if pushing_forward
    % if the grasper is moving forward, need to check if the jaws are
    % closed
    food_moving = grasper_closed_on_food * (1-jaws_closed);
else
    % if grasper is moving backwards, it is assumed the the food is not
    % prevented by the jaws
    food_moving = grasper_closed_on_food;
end

dL_ingested = food_moving * dxf;

== matlab function CMU_BORG_AplysiaModularNeuromechanics/Kinetics and Kinematics1/Kinematics (Circular Odontophore)/Find Dorsal Tangency ==
  data: Xcom input; Xt output size=2; Xa input; R input
function Xt = fcn(Xcom,Xa,R)
% finds the location on the odontophore that forms a tangent line to the
% anchor point at Xa. Xcom is the current center of mass of the odontophore
% with radius R. 


xa = Xa(1) - Xcom(1);
ya = Xa(2) - Xcom(2);



dxt1 = (xa*R^2 + R*ya*sqrt( xa^2 + ya^2 - R^2 )) / ( xa^2 + ya^2 );
dxt2 = (xa*R^2 - R*ya*sqrt( xa^2 + ya^2 - R^2 )) / ( xa^2 + ya^2 );


dxt = min([dxt1,dxt2]);

dyt = (R^2 - xa*dxt)/ya;

Xt = [dxt;dyt] + Xcom;

== matlab function CMU_BORG_AplysiaModularNeuromechanics/Kinetics and Kinematics1/Kinematics (Circular Odontophore)/Find Ventral Tangency ==
  data: Xcom input; Xt output size=2; Xa input; R input
function Xt = fcn(Xcom,Xa,R)
% finds the location on the odontophore that forms a tangent line to the
% anchor point at Xa. Xcom is the current center of mass of the odontophore
% with radius R. 

xa = Xa(1) - Xcom(1);
ya = Xa(2) - Xcom(2);

if (xa^2 + ya^2 < R^2)
    % point is inside the circle
    dxt = xa;
    dyt = -sqrt(R^2 - dxt^2);
else
    dxt1 = (xa*R^2 + R*ya*sqrt( xa^2 + ya^2 - R^2 )) / ( xa^2 + ya^2 );
    dxt2 = (xa*R^2 - R*ya*sqrt( xa^2 + ya^2 - R^2 )) / ( xa^2 + ya^2 );
    
    
    dxt = min([dxt1,dxt2]);
    
    dyt = (R^2 - xa*dxt)/ya;

end
Xt = [dxt;dyt] + Xcom;
